simulink model "MIT_feedforward"  (R2023a)
settings: Solver=FixedStepAuto  StartTime=start_time  StopTime=stop_time  FixedStep=sample_time  RelTol=1e-3
PreLoadFcn:
  | run('example1.m')
values from neighbouring files (symbols this model uses):
  k = 1    [example1.m]
  k0 = 2    [example1.m]
  lambda = Lambda(i)    [example1.m]    (also in example2.m = 1)
  stop_time = 100.0    (= 100)    [Lyapunov_rule_order2.m]    (also in example1.m = 20; example2.m = 500)
settings Model: Creator=Mmoha  LastModifiedBy=Mmoha

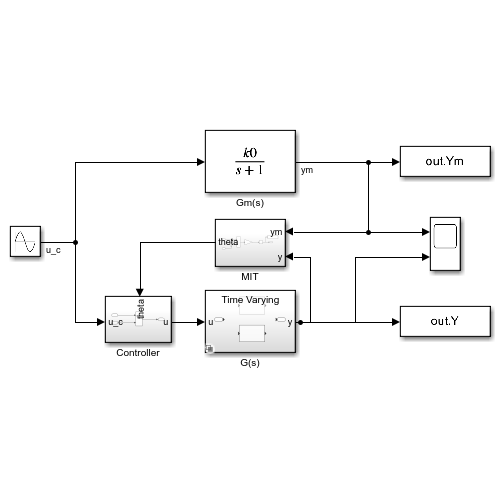
[thumbnail: Simulink's stored preview of the top-level diagram]
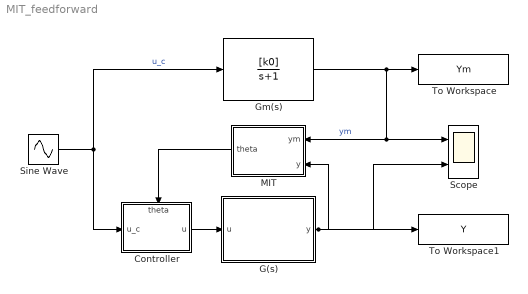
== system MIT_feedforward ==
  Controller : Subsystem
      settings: PortSchema="{\"entries\":[{\"content\":{\"sides\":[{\"content\":{\"connectorIds\":[\"In1\"]},\"type\":\"ConnectorPlacement.EquallySpacedRectSide\",\"uuid\":\"b791fd57-3a4d-44f9-8985-495cef545312\"},{\"content\":{\"connectorIds\":[\"Out1\"],\"side\":\"RIGHT\"},\"type\":\"ConnectorPlacement.EquallySpacedRectSide\",\"uuid\":\"68bf27b1-b1ff-4d62-85c7-49065bb9fd30\"},{\"content\":{\"connectorIds\":[\"In2\"],\"side\":\"TOP\"},\"type\":\"ConnectorPlacement.EquallySpacedRectSide\",\"uuid\":\"5f7f6f71-2cc5-4e24-af1f-d94ef4ac1cd3\"}]},\"type\":\"ConnectorPlacement.EquallySpacedConnector\",\"uuid\":\"a28618e1-4d06-403d-b1b6-c1b4440d8386\"}],\"packageUris\":[\"http://schema.mathworks.com/mf0/Connector/R2020b\"],\"version\":\"1.0\"}"
  G(s) : Subsystem  Variant=on  VariantControlMode=label  VariantControl=Choice  LabelModeActiveChoice=Varying
  Gm(s) : TransferFcn  Numerator=[k0]  Denominator=[1 1]
  MIT : Subsystem
      settings: PortSchema="{\"entries\":[{\"content\":{\"sides\":[{\"content\":{\"connectorIds\":[\"Out1\"]},\"type\":\"ConnectorPlacement.EquallySpacedRectSide\",\"uuid\":\"ee28cc31-6479-493c-b12f-898d8a96a914\"},{\"content\":{\"connectorIds\":[\"In1\",\"In2\"],\"side\":\"RIGHT\"},\"type\":\"ConnectorPlacement.EquallySpacedRectSide\",\"uuid\":\"1e85afc1-68eb-4f3e-8a01-4a66bb1e319d\"},{\"content\":{\"side\":\"TOP\"},\"type\":\"ConnectorPlacement.EquallySpacedRectSide\",\"uuid\":\"df3136a0-60d8-4137-a58e-9a5091616809\"},{\"content\":{\"side\":\"BOTTOM\"},\"type\":\"ConnectorPlacement.EquallySpacedRectSide\",\"uuid\":\"86ec10f5-dbe2-40b7-bc53-b5856bf268b7\"}]},\"type\":\"ConnectorPlacement.EquallySpacedConnector\",\"uuid\":\"e60b5a29-b86c-474a-bd2f-5220248e28cf\"}],\"packageUris\":[\"http://schema.mathworks.com/mf0/Connector/R2020b\"],\"version\":\"1.0\"}"
  Scope : Scope  NumInputPorts=2
  Sine Wave : Sin  SampleTime=0
  To Workspace : ToWorkspace  VariableName=Ym  SaveFormat=Timeseries  SampleTime=-1
  To Workspace1 : ToWorkspace  VariableName=Y  SaveFormat=Timeseries  SampleTime=-1
  wires:
  Sine Wave/1 -> Controller/1(u_c), Gm(s)/1  "u_c"
  Gm(s)/1 -> To Workspace/1, Scope/1, MIT/1(ym)  "ym"
  MIT/1(theta) -> Controller/2(theta)
  Controller/1(u) -> G(s)/1(u)
  G(s)/1(y) -> Scope/2, MIT/2(y), To Workspace1/1

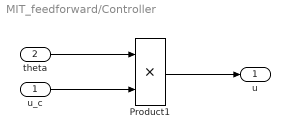
== system MIT_feedforward/Controller ==
  u_c : Inport
  theta : Inport  Port=2
  Product1 : Product
  u : Outport
  wires:
  theta/1 -> Product1/1
  Product1/1 -> u/1
  u_c/1 -> Product1/2

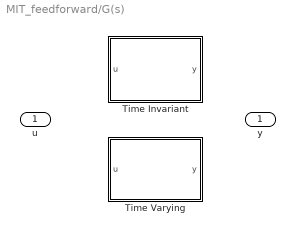
== system MIT_feedforward/G(s) ==
  u : Inport
  Time Invariant : Subsystem  VariantControl=Invariant
  Time Varying : Subsystem  VariantControl=Varying
  y : Outport

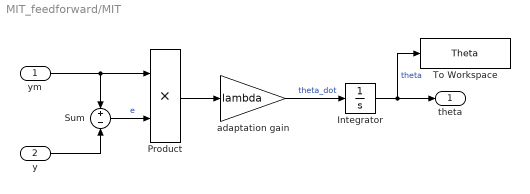
== system MIT_feedforward/MIT ==
  ym : Inport
  y : Inport  Port=2
  Integrator : Integrator
  Product : Product
  Sum : Sum  Inputs=+|-
  To Workspace : ToWorkspace  VariableName=Theta  SaveFormat=Timeseries  SampleTime=-1
  adaptation gain : Gain  Gain=lambda
  theta : Outport
  wires:
  adaptation gain/1 -> Integrator/1  "theta_dot"
  ym/1 -> Product/1, Sum/1
  y/1 -> Sum/2
  Sum/1 -> Product/2  "e"
  Product/1 -> adaptation gain/1
  Integrator/1 -> To Workspace/1, theta/1  "theta"

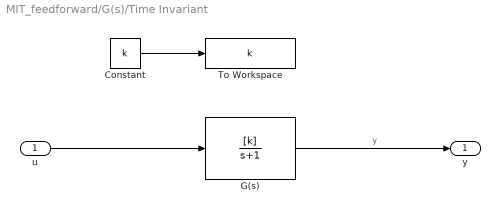
== system MIT_feedforward/G(s)/Time Invariant ==
  u : Inport
  Constant : Constant  Value=k
  G(s) : TransferFcn  Numerator=[k]  Denominator=[1 1]
  To Workspace : ToWorkspace  VariableName=k  SaveFormat=Timeseries  SampleTime=-1
  y : Outport
  wires:
  G(s)/1 -> y/1  "y"
  u/1 -> G(s)/1
  Constant/1 -> To Workspace/1

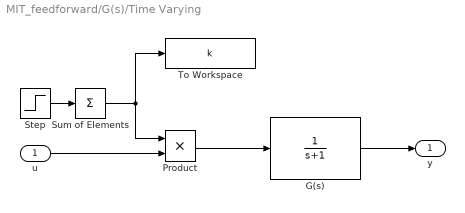
== system MIT_feedforward/G(s)/Time Varying ==
  u : Inport
  G(s) : TransferFcn  Denominator=[1 1]
  Product : Product
  Step : Step  Time=[stop_time/3, stop_time*2/3]  Before=[1 0]  After=[2 -1.5]  SampleTime=0
  Sum of Elements : Sum  Inputs=+
  To Workspace : ToWorkspace  VariableName=k  SaveFormat=Timeseries  SampleTime=-1
  y : Outport
  wires:
  u/1 -> Product/2
  Product/1 -> G(s)/1
  G(s)/1 -> y/1
  Step/1 -> Sum of Elements/1
  Sum of Elements/1 -> To Workspace/1, Product/1
